simulink model "Main"  (R2020a)
settings: Solver=FixedStepAuto  StartTime=0.0  StopTime=6  FixedStep=0.00001  RelTol=1e-3
values from neighbouring files (symbols this model uses):
  A = [1 delta delta^2/2 ... (first row only)    [Main_mat.m]
  V = 0.05    [Main_mat.m]
libraries: simulink x2, Gimbal_Lib x1, dspadpt3 x1
settings Model: Creator=idan  LastModifiedBy=idan

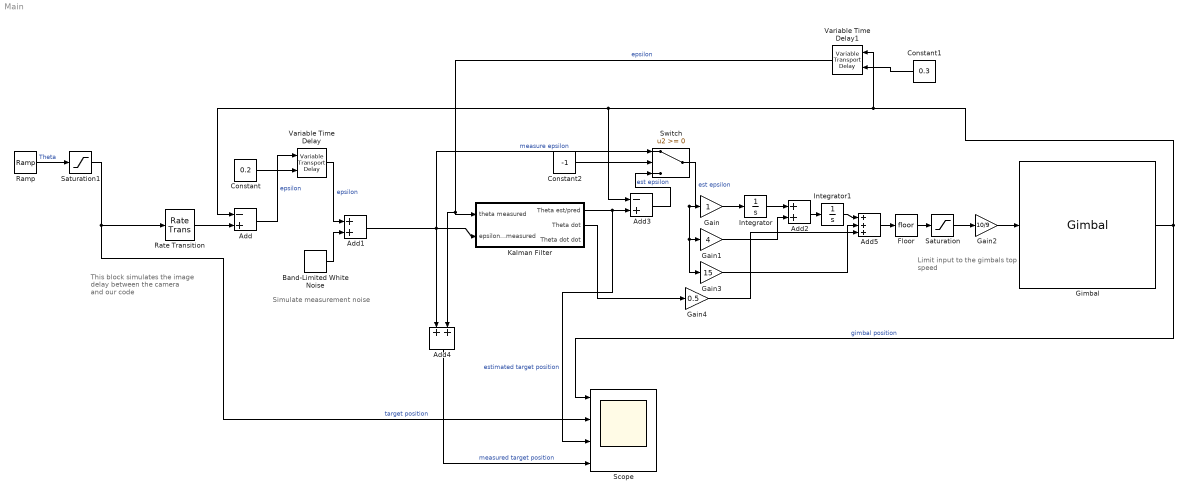
== system Main ==
  note: Simulate measurement noise
  note: Limit input to the
      | gimbals top speed
  note: This block simulates the
      | image delay between the
      | camera and our code
  Add : Sum  Inputs=-+
  Add1 : Sum
  Add2 : Sum
  Add3 : Sum  Inputs=-+
  Add4 : Sum
  Add5 : Sum  Inputs=+++
  Band-Limited White Noise : simulink/Sources/Band-Limited White Noise  Cov=0  Ts=0.1  seed=[23341]
  Constant : Constant  Value=0.2
  Constant1 : Constant  Value=0.3
  Constant2 : Constant  Value=-1
  Floor : Rounding
  Gain : Gain
  Gain1 : Gain  Gain=4
  Gain2 : Gain  Gain=10/9
  Gain3 : Gain  Gain=15
  Gain4 : Gain  Gain=0.5
  Gimbal : Gimbal_Lib/Gimbal  NullSpeedDelay=100
      link override Constant3: Value=0
      link override Edit: Alignment=Center  LabelPosition=Hide
      link override Null Speed Delay: NullSpeedDelay=50
  Integrator : Integrator
  Integrator1 : Integrator
  Kalman Filter : Subsystem
  Ramp : simulink/Sources/Ramp  slope=11.5  start=0.1  InitialOutput=3
  Rate Transition : RateTransition  OutPortSampleTime=1/100
  Saturation : Saturate  UpperLimit=90  LowerLimit=-90
  Saturation1 : Saturate  UpperLimit=40  LowerLimit=-40
  Scope : Scope  NumInputPorts=4
  Switch : Switch
  Variable Time Delay : VariableTransportDelay  MaximumDelay=10  InitialOutput=3
  Variable Time Delay1 : VariableTransportDelay  MaximumDelay=10
  wires:
  Variable Time Delay/1 -> Add1/1  "epsilon"
  Band-Limited White Noise/1 -> Add1/2
  Add1/1 -> Switch/1, Kalman Filter/2(epsilon measured), Add4/1  "measure epsilon"
  Kalman Filter/1(Theta est/pred) -> Scope/3, Add3/2  "estimated target position"
  Gain/1 -> Integrator/1
  Add2/1 -> Integrator1/1
  Rate Transition/1 -> Add/2
  Floor/1 -> Saturation/1
  Saturation/1 -> Gain2/1
  Ramp/1 -> Saturation1/1  "Theta"
  Saturation1/1 -> Rate Transition/1, Scope/2  "target position"
  Constant/1 -> Variable Time Delay/2
  Gimbal/1 -> Add3/1, Add/1, Variable Time Delay1/1, Scope/1  "gimbal position"
  Gain2/1 -> Gimbal/1
  Add/1 -> Variable Time Delay/1  "epsilon"
  Variable Time Delay1/1 -> Add4/2, Kalman Filter/1(theta measured)  "epsilon"
  Constant1/1 -> Variable Time Delay1/2
  Add4/1 -> Scope/4  "measured target position"
  Gain1/1 -> Add2/2
  Integrator/1 -> Add2/1
  Gain3/1 -> Add5/2
  Add5/1 -> Floor/1
  Integrator1/1 -> Add5/1
  Switch/1 -> Gain3/1, Gain1/1, Gain/1  "est epsilon"
  Add3/1 -> Switch/3  "est epsilon"
  Constant2/1 -> Switch/2
  Kalman Filter/2(Theta dot) -> Gain4/1
  Gain4/1 -> Add5/3

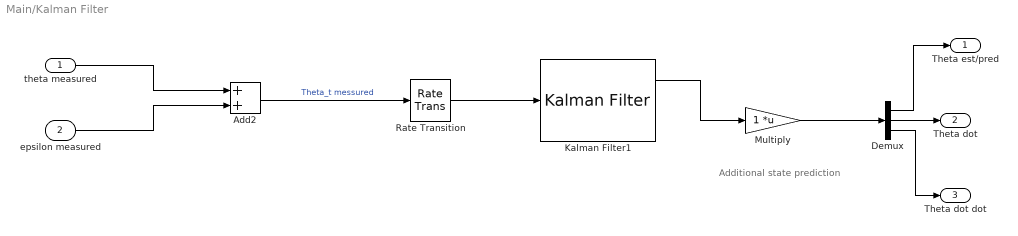
== system Main/Kalman Filter ==
  note: Additional state prediction
  theta measured : Inport
  epsilon measured : Inport  Port=2
  Add2 : Sum
  Demux : Demux  Outputs=3
  Kalman Filter1 : dspadpt3/Kalman Filter  num_targets=1  sourceEnable=Always  isReset=on  X=x_init  P=10*eye(3)  A=A  sourceMeasure=Specify via Dialog  H=C  Q=W  R=V  isOutputEstMeasure=off  isOutputEstState=on  isOutputEstError=off  isOutputPrdMeasure=off  isOutputPrdState=on  isOutputPrdError=off
      settings: SourceProductBaseCode=DS
  Multiply : Gain  Multiplication=Matrix(K*u)
  Rate Transition : RateTransition  OutPortSampleTime=1/100
  Theta est/pred : Outport
  Theta dot : Outport  Port=2
  Theta dot dot : Outport  Port=3
  wires:
  Add2/1 -> Rate Transition/1  "Theta_t messured"
  Demux/3 -> Theta dot dot/1
  Demux/1 -> Theta est/pred/1
  Kalman Filter1/1 -> Multiply/1
  epsilon measured/1 -> Add2/2
  theta measured/1 -> Add2/1
  Demux/2 -> Theta dot/1
  Rate Transition/1 -> Kalman Filter1/1
  Multiply/1 -> Demux/1
